simulink model "Encoder_Position_Detector"  (R2016a)
settings: Solver=VariableStepAuto  StartTime=0.0  StopTime=10.0  RelTol=1e-3
libraries: powerlib_meascontrol x4, simulink x2, dspswit3 x2, simulink_extras x1
settings Model: Creator=ASUS  LastModifiedBy=ASUS

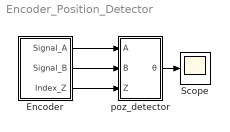
== system Encoder_Position_Detector ==
  Encoder : Subsystem
  Scope : Scope
  poz_detector : Subsystem
  wires:
  Encoder/1(Signal_A) -> poz_detector/1(A)
  Encoder/3(Index_Z) -> poz_detector/3(Z)
  Encoder/2(Signal_B) -> poz_detector/2(B)
  poz_detector/1(θ) -> Scope/1

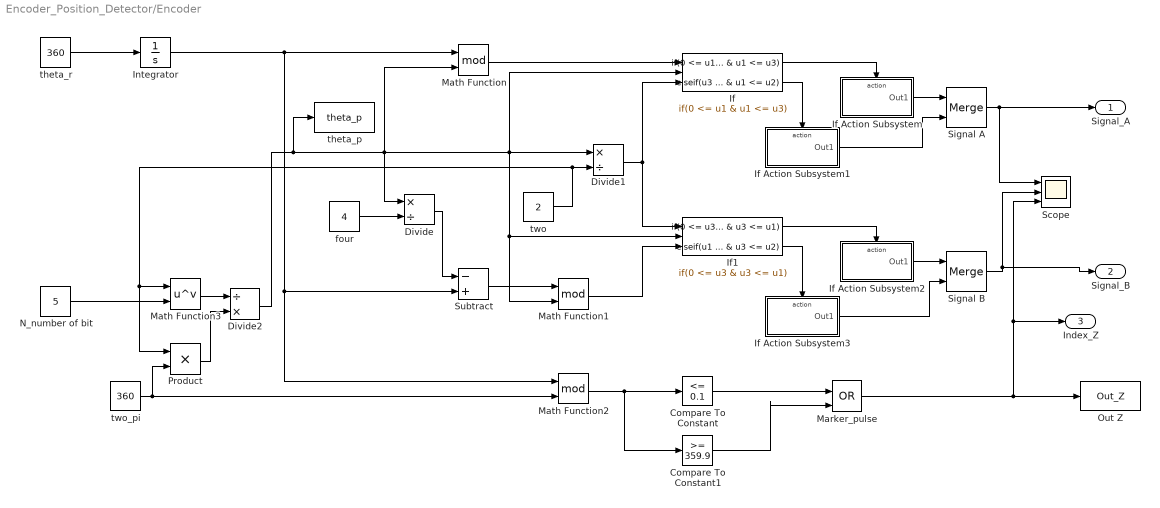
== system Encoder_Position_Detector/Encoder ==
  Compare To Constant : simulink/Logic and Bit Operations/Compare To Constant  relop=<=  const=0.1  OutDataTypeStr=boolean
  Compare To Constant1 : simulink/Logic and Bit Operations/Compare To Constant  relop=>=  const=359.9  OutDataTypeStr=boolean
  Divide : Product  Inputs=*/
  Divide1 : Product  Inputs=*/
  Divide2 : Product  Inputs=/*
  If : If  NumInputs=3  IfExpression=0 <= u1 & u1 <= u3  ElseIfExpressions=u3 < u1 & u1 <= u2  ShowElse=off
  If Action Subsystem : Subsystem  TreatAsAtomicUnit=on
  If Action Subsystem1 : Subsystem  TreatAsAtomicUnit=on
  If Action Subsystem2 : Subsystem  TreatAsAtomicUnit=on
  If Action Subsystem3 : Subsystem  TreatAsAtomicUnit=on
  If1 : If  NumInputs=3  IfExpression=0 <= u3 & u3 <= u1  ElseIfExpressions=u1 < u3 & u3 <= u2  ShowElse=off
  Integrator : Integrator
  Marker_pulse : Logic  Operator=OR  IconShape=distinctive  AllPortsSameDT=off  OutDataTypeStr=boolean
  Math Function : Math  Operator=mod  SaturateOnIntegerOverflow=on
  Math Function1 : Math  Operator=mod  SaturateOnIntegerOverflow=on
  Math Function2 : Math  Operator=mod  SaturateOnIntegerOverflow=on
  Math Function3 : Math  Operator=pow  SaturateOnIntegerOverflow=on
  N_number of bit : Constant  Value=5
  Out Z : ToWorkspace  VariableName=Out_Z  SaveFormat=Timeseries  SampleTime=-1
  Product : Product
  Scope : Scope  NumInputPorts=3
  Signal A : Merge
  Signal B : Merge
  Subtract : Sum  Inputs=-+
  "four " : Constant  Value=4
  theta_p : ToWorkspace  VariableName=theta_p  SaveFormat=Timeseries  SampleTime=-1
  theta_r : Constant  Value=360
  "two " : Constant  Value=2
  "two_pi " : Constant  Value=360
  Signal_A : Outport
  Signal_B : Outport  Port=2
  Index_Z : Outport  Port=3
  wires:
  "two "/1 -> Product/1, Math Function3/1, Divide1/2
  If/1 -> If Action Subsystem/Action
  If Action Subsystem2/1(Out1) -> Signal B/1
  If Action Subsystem1/1(Out1) -> Signal A/2
  Integrator/1 -> Math Function2/1, Subtract/2, Math Function/1
  "four "/1 -> Divide/2
  Divide2/1 -> theta_p/1, Divide/1, Math Function/2, Math Function1/2, If1/2, If/2, Divide1/1
  If Action Subsystem3/1(Out1) -> Signal B/2
  If Action Subsystem/1(Out1) -> Signal A/1
  If/2 -> If Action Subsystem1/Action
  Divide1/1 -> If1/1, If/3
  Math Function1/1 -> If1/3
  Divide/1 -> Subtract/1
  Signal B/1 -> Signal_B/1, Scope/2
  Math Function/1 -> If/1
  Subtract/1 -> Math Function1/1
  Math Function3/1 -> Divide2/1
  Marker_pulse/1 -> Out Z/1, Index_Z/1, Scope/3
  Compare To Constant/1 -> Marker_pulse/1
  Compare To Constant1/1 -> Marker_pulse/2
  N_number of bit/1 -> Math Function3/2
  Product/1 -> Divide2/2
  If1/1 -> If Action Subsystem2/Action
  Math Function2/1 -> Compare To Constant1/1, Compare To Constant/1
  Signal A/1 -> Signal_A/1, Scope/1
  If1/2 -> If Action Subsystem3/Action
  theta_r/1 -> Integrator/1
  "two_pi "/1 -> Product/2, Math Function2/2

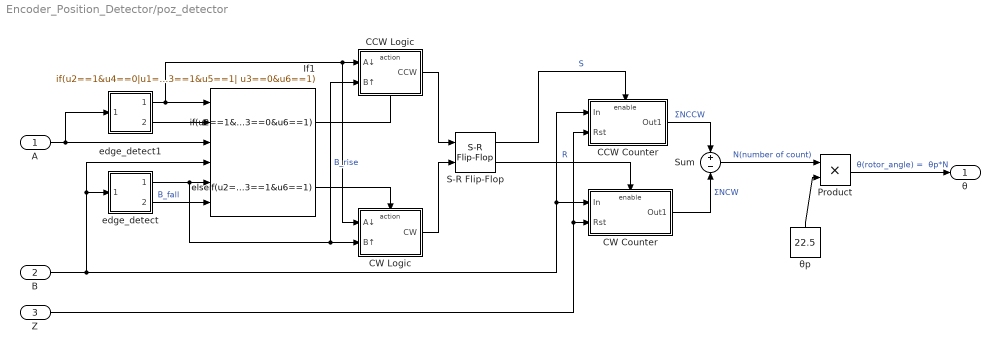
== system Encoder_Position_Detector/poz_detector ==
  A : Inport
  B : Inport  Port=2
  Z : Inport  Port=3
  " θp" : Constant  Value=22.5
  CCW Counter : Subsystem  TreatAsAtomicUnit=on
  CCW Logic : Subsystem  TreatAsAtomicUnit=on
  CW Counter : Subsystem  TreatAsAtomicUnit=on
  CW Logic : Subsystem  TreatAsAtomicUnit=on
  If1 : If  NumInputs=6  IfExpression=u2==1&u4==0|u1==1&u4==1| u3==1&u5==1| u3==0&u6==1  ElseIfExpressions=u2==1&u4==1| u1==1&u4==0 | u3==0&u5==1 | u3==1&u6==1  ShowElse=off
  Product : Product
  S-R Flip-Flop : simulink_extras/Flip Flops/S-R Flip-Flop  initial_condition=0
  Sum : Sum  Inputs=+-
  edge_detect : Subsystem
  edge_detect1 : Subsystem
  θ : Outport
  wires:
  edge_detect/1(B↑) -> CW Logic/2(B↑), CCW Logic/2(B↑), If1/5  "B_rise"
  " θp"/1 -> Product/2
  A/1 -> If1/3, edge_detect1/1(In1)
  Z/1 -> CW Counter/2(Rst), CCW Counter/2(Rst)
  If1/1 -> CCW Logic/Action
  B/1 -> CCW Counter/1(In), CW Counter/1(In), If1/4, edge_detect/1(In1)
  S-R Flip-Flop/1 -> CCW Counter/Enable  "S"
  S-R Flip-Flop/2 -> CW Counter/Enable  "R"
  CCW Counter/1(Out1) -> Sum/1  "ΣNCCW"
  CW Counter/1(Out1) -> Sum/2  "ΣNCW"
  Sum/1 -> Product/1  "N(number of count)"
  Product/1 -> θ/1  "θ(rotor_angle) =  θp*N"
  edge_detect/2(B↓) -> If1/6  "B_fall"
  CW Logic/1(CW) -> S-R Flip-Flop/2
  If1/2 -> CW Logic/Action
  edge_detect1/2(A↑) -> If1/2
  CCW Logic/1(CCW) -> S-R Flip-Flop/1
  edge_detect1/1(A↓) -> CW Logic/1(A↓), CCW Logic/1(A↓), If1/1

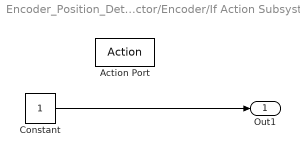
== system Encoder_Position_Detector/Encoder/If Action Subsystem ==
  Action Port : ActionPort  ActionType=then
  Constant : Constant
  Out1 : Outport
  wires:
  Constant/1 -> Out1/1

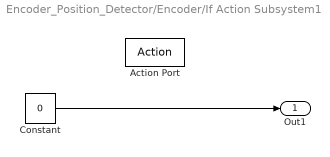
== system Encoder_Position_Detector/Encoder/If Action Subsystem1 ==
  Action Port : ActionPort  ActionType=elseif
  Constant : Constant  Value=0
  Out1 : Outport
  wires:
  Constant/1 -> Out1/1

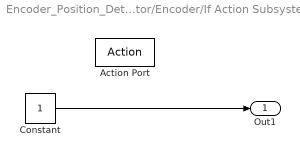
== system Encoder_Position_Detector/Encoder/If Action Subsystem2 ==
  Action Port : ActionPort  ActionType=then
  Constant : Constant
  Out1 : Outport
  wires:
  Constant/1 -> Out1/1

== system Encoder_Position_Detector/Encoder/If Action Subsystem3 ==
  Action Port : ActionPort  ActionType=elseif
  Constant : Constant  Value=0
  Out1 : Outport
  wires:
  Constant/1 -> Out1/1

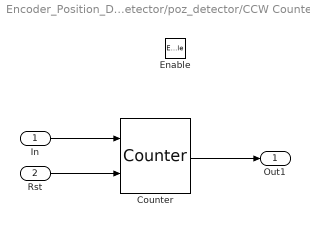
== system Encoder_Position_Detector/poz_detector/CCW Counter ==
  In : Inport
  Rst : Inport  Port=2
  Enable : EnablePort
  Counter : dspswit3/Counter  Direction=Up  CountEvent=Rising edge  CounterSize=User defined  MaxCount=255  InitialCount=0  Output=Count  HitValue=32  ResetInput=on  SamplesPerFrame=1  Ts=1  CntDtype=double  HitDtype=Logical
  Out1 : Outport
  wires:
  In/1 -> Counter/1
  Rst/1 -> Counter/2
  Counter/1 -> Out1/1

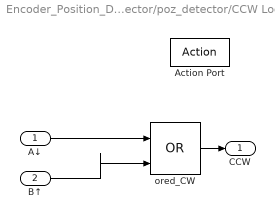
== system Encoder_Position_Detector/poz_detector/CCW Logic ==
  A↓ : Inport
  B↑ : Inport  Port=2
  Action Port : ActionPort  ActionType=then
  ored_CW : Logic  Operator=OR  IconShape=distinctive  AllPortsSameDT=off  OutDataTypeStr=boolean
  CCW : Outport
  wires:
  A↓/1 -> ored_CW/1
  B↑/1 -> ored_CW/2
  ored_CW/1 -> CCW/1

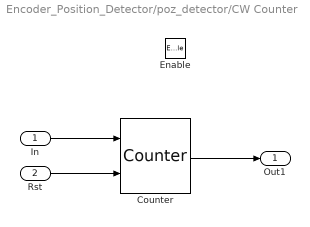
== system Encoder_Position_Detector/poz_detector/CW Counter ==
  In : Inport
  Rst : Inport  Port=2
  Enable : EnablePort
  Counter : dspswit3/Counter  Direction=Up  CountEvent=Rising edge  CounterSize=User defined  MaxCount=255  InitialCount=0  Output=Count  HitValue=32  ResetInput=on  SamplesPerFrame=1  Ts=1  CntDtype=double  HitDtype=Logical
  Out1 : Outport
  wires:
  In/1 -> Counter/1
  Rst/1 -> Counter/2
  Counter/1 -> Out1/1

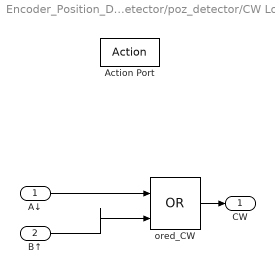
== system Encoder_Position_Detector/poz_detector/CW Logic ==
  A↓ : Inport
  B↑ : Inport  Port=2
  Action Port : ActionPort  ActionType=elseif
  ored_CW : Logic  Operator=OR  IconShape=distinctive  AllPortsSameDT=off  OutDataTypeStr=boolean
  CW : Outport
  wires:
  A↓/1 -> ored_CW/1
  B↑/1 -> ored_CW/2
  ored_CW/1 -> CW/1

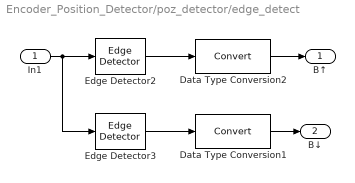
== system Encoder_Position_Detector/poz_detector/edge_detect ==
  In1 : Inport
  Data Type Conversion1 : DataTypeConversion
  Data Type Conversion2 : DataTypeConversion
  Edge Detector2 : powerlib_meascontrol/Logic/Edge Detector  model=Rising  ic=0  Ts=0
  Edge Detector3 : powerlib_meascontrol/Logic/Edge Detector  model=Falling  ic=0  Ts=0
  B↑ : Outport
  B↓ : Outport  Port=2
  wires:
  In1/1 -> Edge Detector3/1, Edge Detector2/1
  Edge Detector2/1 -> Data Type Conversion2/1
  Edge Detector3/1 -> Data Type Conversion1/1
  Data Type Conversion2/1 -> B↑/1
  Data Type Conversion1/1 -> B↓/1

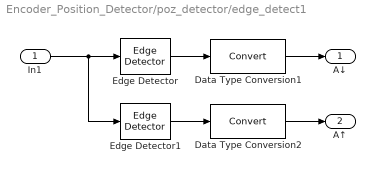
== system Encoder_Position_Detector/poz_detector/edge_detect1 ==
  In1 : Inport
  Data Type Conversion1 : DataTypeConversion
  Data Type Conversion2 : DataTypeConversion
  Edge Detector : powerlib_meascontrol/Logic/Edge Detector  model=Falling  ic=0  Ts=0
  Edge Detector1 : powerlib_meascontrol/Logic/Edge Detector  model=Rising  ic=0  Ts=0
  A↓ : Outport
  A↑ : Outport  Port=2
  wires:
  In1/1 -> Edge Detector1/1, Edge Detector/1
  Edge Detector/1 -> Data Type Conversion1/1
  Edge Detector1/1 -> Data Type Conversion2/1
  Data Type Conversion1/1 -> A↓/1
  Data Type Conversion2/1 -> A↑/1
